simulink model "DA42HoloLensForwarder"  (R2021a)
settings: Solver=ode4  StartTime=0.0  StopTime=inf  FixedStep=0.001  RelTol=1e-3
undefined symbols (not defined in the file): Global_Sample_Time
libraries: simulink_extras x5, slrealtimeutilitieslib x2, dspnetwork x1
(part 1 of 5)
settings Model: EnablePacing=on  Creator=FCS Lab  LastModifiedBy=ga28nex
settings SolverCC: AlgebraicLoopSolver=TrustRegion
settings DebuggingCC: SFMachineParentedDataDiag=warning

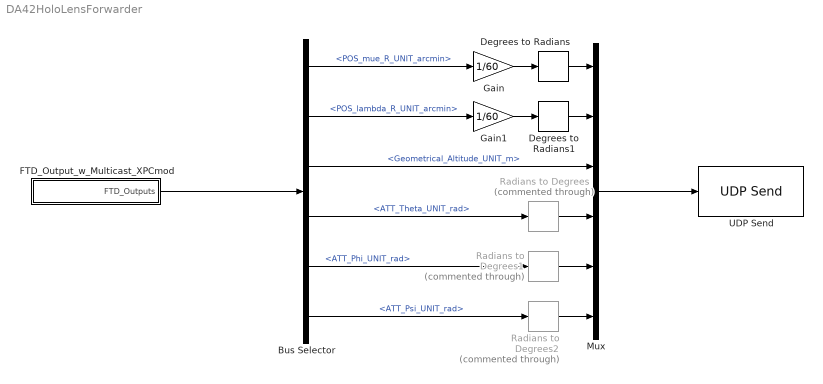
== system DA42HoloLensForwarder ==
  Bus Selector : BusSelector  OutputSignals=Host_Signals.POS_mue_R_UNIT_arcmin,Host_Signals.POS_lambda_R_UNIT_arcmin,Host_Signals.Geometrical_Altitude_UNIT_m,Host_Signals.ATT_Theta_UNIT_rad,Host_Signals.ATT_Phi_UNIT_rad,Host_Signals.ATT_Psi_UNIT_rad
  Degrees to Radians : simulink_extras/Transformations/Degrees to Radians
  Degrees to Radians1 : simulink_extras/Transformations/Degrees to Radians
  FTD_Output_w_Multicast_XPCmod : Subsystem
  Gain : Gain  Gain=1/60
  Gain1 : Gain  Gain=1/60
  Mux : Mux  Inputs=6
  Radians to Degrees : simulink_extras/Transformations/Radians to Degrees  Commented=through
  Radians to Degrees1 : simulink_extras/Transformations/Radians to Degrees  Commented=through
  Radians to Degrees2 : simulink_extras/Transformations/Radians to Degrees  Commented=through
  UDP Send : dspnetwork/UDP Send  remoteURL='127.0.0.1'  remotePort=53941  localURL='0.0.0.0'  localPortSource=Automatically determine  localPort=-1  sendBufferSize=8192  sampletime=-1  blockPlatform=[]  separateLengthPort=0
  wires:
  FTD_Output_w_Multicast_XPCmod/1(FTD_Outputs) -> Bus Selector/1
  Bus Selector/1 -> Gain/1  "<POS_mue_R_UNIT_arcmin>"
  Bus Selector/2 -> Gain1/1  "<POS_lambda_R_UNIT_arcmin>"
  Bus Selector/3 -> Mux/3  "<Geometrical_Altitude_UNIT_m>"
  Radians to Degrees/1 -> Mux/4
  Bus Selector/4 -> Radians to Degrees/1  "<ATT_Theta_UNIT_rad>"
  Radians to Degrees1/1 -> Mux/5
  Bus Selector/5 -> Radians to Degrees1/1  "<ATT_Phi_UNIT_rad>"
  Radians to Degrees2/1 -> Mux/6
  Bus Selector/6 -> Radians to Degrees2/1  "<ATT_Psi_UNIT_rad>"
  Mux/1 -> UDP Send/1
  Gain1/1 -> Degrees to Radians1/1
  Gain/1 -> Degrees to Radians/1
  Degrees to Radians/1 -> Mux/1
  Degrees to Radians1/1 -> Mux/2

== system DA42HoloLensForwarder/FTD_Output_w_Multicast_XPCmod ==
  Bus Creator : BusCreator  Inputs=3
  Hardware_Switches : Subsystem
  Host_Signals : Subsystem
  IO_Module_Pilot_Commands : Subsystem
  FTD_Outputs : Outport  BusOutputAsStruct=on
  wires:
  Bus Creator/1 -> FTD_Outputs/1  "FTD_Outputs"
  Host_Signals/1(Host_Signals) -> Bus Creator/1
  Hardware_Switches/1(Hardware_Switches) -> Bus Creator/3
  IO_Module_Pilot_Commands/1(Commands_Bus) -> Bus Creator/2
  IO_Module_Pilot_Commands/2(Switches) -> Hardware_Switches/1(Switches)

== system DA42HoloLensForwarder/FTD_Output_w_Multicast_XPCmod/Hardware_Switches ==
  note: CVCLVariable<double> MiscSwitches;
      | 	CVCLVariable<double> PanelAndLegroomSwitches;
      | 	CVCLVariable<double> SticksAndConsoleSwitches;
      | 	CVCLVariable<double> SticksDeviceConsoleSwitches;
  Switches : Inport
  Bus Creator2 : BusCreator  Inputs=3  NonVirtualBus=on
  Bus Selector : BusSelector  OutputSignals=MiscSwitches,PanelAndLegroomSwitches,SticksAndConsoleSwitches
  MiscSwitches : Subsystem
  PanelAndLegroomSwitches : Subsystem
  SticksAndConsoleSwitches : Subsystem
  Hardware_Switches : Outport
  wires:
  Bus Selector/2 -> PanelAndLegroomSwitches/1(PanelAndLegroomSwitches_MASK)  "<PanelAndLegroomSwitches>"
  Bus Selector/1 -> MiscSwitches/1(PanelAndLegroomSwitches_MASK)  "<MiscSwitches>"
  Bus Selector/3 -> SticksAndConsoleSwitches/1(PanelAndLegroomSwitches_MASK)  "<SticksAndConsoleSwitches>"
  PanelAndLegroomSwitches/1(PanelAndLegroomSwitches) -> Bus Creator2/2
  Bus Creator2/1 -> Hardware_Switches/1  "Hardware_Switches"
  MiscSwitches/1(MiscSwitches) -> Bus Creator2/1
  SticksAndConsoleSwitches/1(SticksAndConsoleSwitches) -> Bus Creator2/3
  Switches/1 -> Bus Selector/1

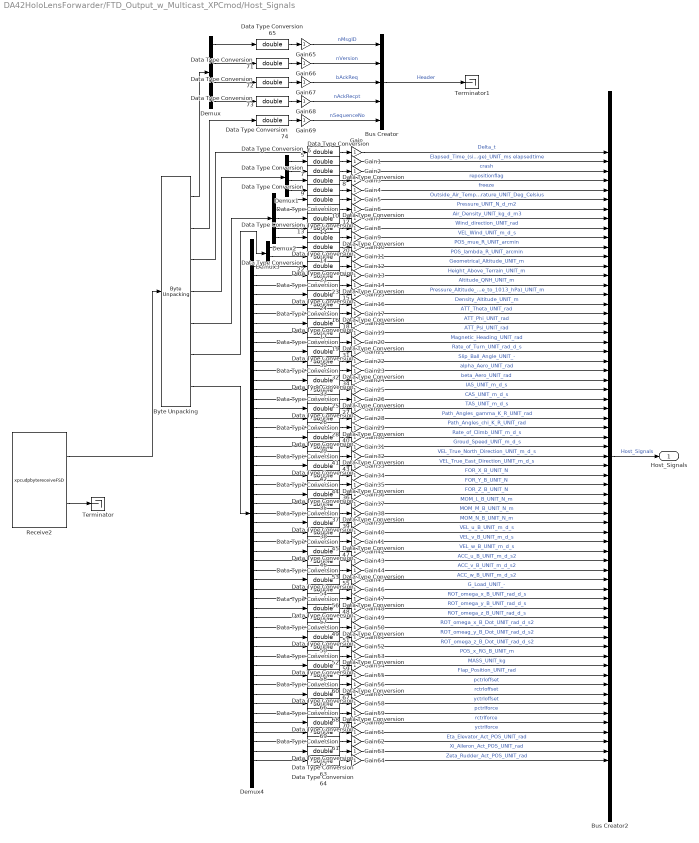
== system DA42HoloLensForwarder/FTD_Output_w_Multicast_XPCmod/Host_Signals ==
  Bus Creator : BusCreator  Inputs=5
  Bus Creator2 : BusCreator  Inputs=65  NonVirtualBus=on
  "Byte Unpacking " : slrealtimeutilitieslib/Byte Unpacking  MaskUnpackedDataTypes="{'uint8', 'uint32', 'single',  'uint32', 'single', 'double', 'single'}"  MaskUnpackedDataSizes={4, 1, 1, 4, 5, 2, 53}  MaskAlignment=1
      settings: SourceProductBaseCode=XP
  Data Type Conversion{5..74} (70 alike) : DataTypeConversion  OutDataTypeStr=double
  Demux : Demux
  Demux1 : Demux
  Demux2 : Demux  Outputs=5
  Demux3 : Demux  Outputs=2
  Demux4 : Demux  Outputs=53
  Gain{,1..69} (70 alike) : Gain
  Receive2 : S-Function  FunctionName=xpcudpbytereceiveFSD  Parameters=ipAdd, ipPort, width, sampletime, vblLen  SFunctionDeploymentMode=off  EnableBusSupport=off  mask(xpcudpbytereceive){ipAddress=234.1.1.2, ipPort=15150, width=276, vblLen=on, sampletime=Global_Sample_Time}
      mask prompts: ipAddress "IP address to receive from (0.0.0.0 for accepting all):"; ipPort "IP port to receive from:"; width "Output port width (number of bytes):"; vblLen "Allow variable length packets"; sampletime "Sample time:"
      mask init:
      | % mudp('ipPort', 'IP Port');
      | ipAdd = ipAddressFromString(ipAddress);
      mask Help: eval('xpcdoc(''UDP_Receive'')');
      mask Display: disp('FSD\nUDP-Receive\nBinary')
  Terminator : Terminator
  Terminator1 : Terminator
  Host_Signals : Outport
  wires:
  Receive2/2 -> Terminator/1
  Receive2/1 -> "Byte Unpacking "/1
  Gain64/1 -> Bus Creator2/65  "Zeta_Rudder_Act_POS_UNIT_rad"
  Gain63/1 -> Bus Creator2/64  "Xi_Aileron_Act_POS_UNIT_rad"
  Gain62/1 -> Bus Creator2/63  "Eta_Elevator_Act_POS_UNIT_rad"
  Gain61/1 -> Bus Creator2/62  "yctrlforce"
  Gain60/1 -> Bus Creator2/61  "rctrlforce"
  Gain59/1 -> Bus Creator2/60  "pctrlforce"
  Gain58/1 -> Bus Creator2/59  "yctrloffset"
  Gain57/1 -> Bus Creator2/58  "rctrloffset"
  Gain56/1 -> Bus Creator2/57  "pctrloffset"
  Gain55/1 -> Bus Creator2/56  "Flap_Position_UNIT_rad"
  Gain54/1 -> Bus Creator2/55  "MASS_UNIT_kg"
  Gain53/1 -> Bus Creator2/54  "POS_x_RG_B_UNIT_m"
  Gain52/1 -> Bus Creator2/53  "ROT_omega_z_B_Dot_UNIT_rad_d_s2"
  Gain51/1 -> Bus Creator2/52  "ROT_omeag_y_B_Dot_UNIT_rad_d_s2"
  Gain50/1 -> Bus Creator2/51  "ROT_omega_x_B_Dot_UNIT_rad_d_s2"
  Gain49/1 -> Bus Creator2/50  "ROT_omega_z_B_UNIT_rad_d_s"
  Gain48/1 -> Bus Creator2/49  "ROT_omega_y_B_UNIT_rad_d_s"
  Gain47/1 -> Bus Creator2/48  "ROT_omega_x_B_UNIT_rad_d_s"
  Gain46/1 -> Bus Creator2/47  "G_Load_UNIT_-"
  Gain45/1 -> Bus Creator2/46  "ACC_w_B_UNIT_m_d_s2"
  Gain44/1 -> Bus Creator2/45  "ACC_v_B_UNIT_m_d_s2"
  Gain43/1 -> Bus Creator2/44  "ACC_u_B_UNIT_m_d_s2"
  Gain42/1 -> Bus Creator2/43  "VEL_w_B_UNIT_m_d_s"
  Gain41/1 -> Bus Creator2/42  "VEL_v_B_UNIT_m_d_s"
  Gain40/1 -> Bus Creator2/41  "VEL_u_B_UNIT_m_d_s"
  Gain39/1 -> Bus Creator2/40  "MOM_N_B_UNIT_N_m"
  Gain38/1 -> Bus Creator2/39  "MOM_M_B_UNIT_N_m"
  Gain37/1 -> Bus Creator2/38  "MOM_L_B_UNIT_N_m"
  Gain36/1 -> Bus Creator2/37  "FOR_Z_B_UNIT_N"
  Gain35/1 -> Bus Creator2/36  "FOR_Y_B_UNIT_N"
  Gain34/1 -> Bus Creator2/35  "FOR_X_B_UNIT_N"
  Gain33/1 -> Bus Creator2/34  "VEL_True_East_Direction_UNIT_m_d_s"
  Gain32/1 -> Bus Creator2/33  "VEL_True_North_Direction_UNIT_m_d_s"
  Gain31/1 -> Bus Creator2/32  "Groud_Speed_UNIT_m_d_s"
  Gain30/1 -> Bus Creator2/31  "Rate_of_Climb_UNIT_m_d_s"
  Gain29/1 -> Bus Creator2/30  "Path_Angles_chi_K_R_UNIT_rad"
  Gain28/1 -> Bus Creator2/29  "Path_Angles_gamma_K_R_UNIT_rad"
  Gain27/1 -> Bus Creator2/28  "TAS_UNIT_m_d_s"
  Gain26/1 -> Bus Creator2/27  "CAS_UNIT_m_d_s"
  Gain25/1 -> Bus Creator2/26  "IAS_UNIT_m_d_s"
  Gain24/1 -> Bus Creator2/25  "beta_Aero_UNIT_rad"
  Bus Creator2/1 -> Host_Signals/1  "Host_Signals"
  Gain23/1 -> Bus Creator2/24  "alpha_Aero_UNIT_rad"
  Gain22/1 -> Bus Creator2/23  "Slip_Ball_Angle_UNIT_-"
  Gain21/1 -> Bus Creator2/22  "Rate_of_Turn_UNIT_rad_d_s"
  Gain20/1 -> Bus Creator2/21  "Magnetic_Heading_UNIT_rad"
  Gain19/1 -> Bus Creator2/20  "ATT_Psi_UNIT_rad"
  Gain18/1 -> Bus Creator2/19  "ATT_Phi_UNIT_rad"
  Gain17/1 -> Bus Creator2/18  "ATT_Theta_UNIT_rad"
  Gain16/1 -> Bus Creator2/17  "Density_Altitude_UNIT_m"
  Gain15/1 -> Bus Creator2/16  "Pressure_Altitude_(relative_to_1013_hPa)_UNIT_m"
  Gain14/1 -> Bus Creator2/15  "Altitude_QNH_UNIT_m"
  Gain13/1 -> Bus Creator2/14  "Height_Above_Terrain_UNIT_m"
  Gain12/1 -> Bus Creator2/13  "Geometrical_Altitude_UNIT_m"
  Gain11/1 -> Bus Creator2/12  "POS_lambda_R_UNIT_arcmin"
  Gain10/1 -> Bus Creator2/11  "POS_mue_R_UNIT_arcmin"
  Gain9/1 -> Bus Creator2/10  "VEL_Wind_UNIT_m_d_s"
  Gain8/1 -> Bus Creator2/9  "Wind_direction_UNIT_rad"
  Gain7/1 -> Bus Creator2/8  "Air_Density_UNIT_kg_d_m3"
  Gain6/1 -> Bus Creator2/7  "Pressure_UNIT_N_d_m2"
  Gain5/1 -> Bus Creator2/6  "Outside_Air_Temperature_UNIT_Deg_Celsius"
  Gain4/1 -> Bus Creator2/5  "freeze"
  Gain3/1 -> Bus Creator2/4  "repositionflag"
  Gain2/1 -> Bus Creator2/3  "crash"
  Gain1/1 -> Bus Creator2/2  "Elapsed_Time_(since_last_time_change)_UNIT_ms elapsedtime"
  Gain/1 -> Bus Creator2/1  "Delta_t"
  Data Type Conversion5/1 -> Gain/1
  Data Type Conversion6/1 -> Gain1/1
  Data Type Conversion7/1 -> Gain2/1
  Data Type Conversion8/1 -> Gain3/1
  Data Type Conversion9/1 -> Gain4/1
  Data Type Conversion10/1 -> Gain5/1
  Data Type Conversion11/1 -> Gain6/1
  Data Type Conversion12/1 -> Gain7/1
  Data Type Conversion13/1 -> Gain8/1
  Data Type Conversion14/1 -> Gain9/1
  Data Type Conversion20/1 -> Gain10/1
  Data Type Conversion21/1 -> Gain11/1
  Data Type Conversion22/1 -> Gain12/1
  Data Type Conversion23/1 -> Gain13/1
  Data Type Conversion24/1 -> Gain14/1
  Data Type Conversion15/1 -> Gain15/1
  Data Type Conversion16/1 -> Gain16/1
  Data Type Conversion17/1 -> Gain17/1
  Data Type Conversion18/1 -> Gain18/1
  Data Type Conversion19/1 -> Gain19/1
  Data Type Conversion30/1 -> Gain20/1
  Data Type Conversion31/1 -> Gain21/1
  Data Type Conversion32/1 -> Gain22/1
  Data Type Conversion33/1 -> Gain23/1
  Data Type Conversion34/1 -> Gain24/1
  Data Type Conversion25/1 -> Gain25/1
  Data Type Conversion26/1 -> Gain26/1
  Data Type Conversion27/1 -> Gain27/1
  Data Type Conversion28/1 -> Gain28/1
  Data Type Conversion29/1 -> Gain29/1
  Data Type Conversion40/1 -> Gain30/1
  Data Type Conversion41/1 -> Gain31/1
  Data Type Conversion42/1 -> Gain32/1
  Data Type Conversion43/1 -> Gain33/1
  Data Type Conversion44/1 -> Gain34/1
  Data Type Conversion35/1 -> Gain35/1
  Data Type Conversion36/1 -> Gain36/1
  Data Type Conversion37/1 -> Gain37/1
  Data Type Conversion38/1 -> Gain38/1
  Data Type Conversion39/1 -> Gain39/1
  Data Type Conversion45/1 -> Gain40/1
  Data Type Conversion46/1 -> Gain41/1
  Data Type Conversion47/1 -> Gain42/1
  Data Type Conversion53/1 -> Gain43/1
  Data Type Conversion54/1 -> Gain44/1
  Data Type Conversion55/1 -> Gain45/1
  Data Type Conversion56/1 -> Gain46/1
  Data Type Conversion57/1 -> Gain47/1
  Data Type Conversion48/1 -> Gain48/1
  Data Type Conversion49/1 -> Gain49/1
  Data Type Conversion50/1 -> Gain50/1
  Data Type Conversion51/1 -> Gain51/1
  Data Type Conversion52/1 -> Gain52/1
  Data Type Conversion58/1 -> Gain53/1
  Data Type Conversion59/1 -> Gain54/1
  Data Type Conversion60/1 -> Gain55/1
  Data Type Conversion66/1 -> Gain56/1
  Data Type Conversion67/1 -> Gain57/1
  Data Type Conversion68/1 -> Gain58/1
  Data Type Conversion69/1 -> Gain59/1
  Data Type Conversion70/1 -> Gain60/1
  Data Type Conversion61/1 -> Gain61/1
  Data Type Conversion62/1 -> Gain62/1
  Data Type Conversion63/1 -> Gain63/1
  Data Type Conversion64/1 -> Gain64/1
  "Byte Unpacking "/1 -> Demux/1
  "Byte Unpacking "/4 -> Demux1/1
  "Byte Unpacking "/5 -> Demux2/1
  "Byte Unpacking "/6 -> Demux3/1
  "Byte Unpacking "/7 -> Demux4/1
  Demux4/1 -> Data Type Conversion22/1
  Demux4/2 -> Data Type Conversion23/1
  Demux4/3 -> Data Type Conversion24/1
  Demux4/4 -> Data Type Conversion15/1
  Demux4/5 -> Data Type Conversion16/1
  Demux4/6 -> Data Type Conversion17/1
  Demux4/7 -> Data Type Conversion18/1
  Demux4/8 -> Data Type Conversion19/1
  Demux4/9 -> Data Type Conversion30/1
  Demux4/10 -> Data Type Conversion31/1
  Demux4/11 -> Data Type Conversion32/1
  Demux4/12 -> Data Type Conversion33/1
  Demux4/13 -> Data Type Conversion34/1
  Demux4/14 -> Data Type Conversion25/1
  Demux4/15 -> Data Type Conversion26/1
  Demux4/16 -> Data Type Conversion27/1
  Demux4/17 -> Data Type Conversion28/1
  Demux4/18 -> Data Type Conversion29/1
  Demux4/19 -> Data Type Conversion40/1
  Demux4/20 -> Data Type Conversion41/1
  Demux4/21 -> Data Type Conversion42/1
  Demux4/22 -> Data Type Conversion43/1
  Demux4/23 -> Data Type Conversion44/1
  Demux4/24 -> Data Type Conversion35/1
  Demux4/25 -> Data Type Conversion36/1
  Demux4/26 -> Data Type Conversion37/1
  Demux4/27 -> Data Type Conversion38/1
  Demux4/28 -> Data Type Conversion39/1
  Demux4/29 -> Data Type Conversion45/1
  Demux4/30 -> Data Type Conversion46/1
  Demux4/31 -> Data Type Conversion47/1
  Demux4/32 -> Data Type Conversion53/1
  Demux4/33 -> Data Type Conversion54/1
  Demux4/34 -> Data Type Conversion55/1
  Demux4/35 -> Data Type Conversion56/1
  Demux4/36 -> Data Type Conversion57/1
  Demux4/37 -> Data Type Conversion48/1
  Demux4/38 -> Data Type Conversion49/1
  Demux4/39 -> Data Type Conversion50/1
  Demux4/40 -> Data Type Conversion51/1
  Demux4/41 -> Data Type Conversion52/1
  Demux4/42 -> Data Type Conversion58/1
  Demux4/43 -> Data Type Conversion59/1
  Demux4/44 -> Data Type Conversion60/1
  Demux4/45 -> Data Type Conversion66/1
  Demux4/46 -> Data Type Conversion67/1
  Demux4/47 -> Data Type Conversion68/1
  Demux4/48 -> Data Type Conversion69/1
  Demux4/49 -> Data Type Conversion70/1
  Demux4/50 -> Data Type Conversion61/1
  Demux4/51 -> Data Type Conversion62/1
  Demux4/52 -> Data Type Conversion63/1
  Demux4/53 -> Data Type Conversion64/1
  Demux3/1 -> Data Type Conversion20/1
  Demux3/2 -> Data Type Conversion21/1
  Demux2/1 -> Data Type Conversion10/1
  Demux2/2 -> Data Type Conversion11/1
  Demux2/3 -> Data Type Conversion12/1
  Demux2/4 -> Data Type Conversion13/1
  Demux2/5 -> Data Type Conversion14/1
  Demux1/1 -> Data Type Conversion6/1
  Demux1/2 -> Data Type Conversion7/1
  Demux1/3 -> Data Type Conversion8/1
  Demux1/4 -> Data Type Conversion9/1
  "Byte Unpacking "/3 -> Data Type Conversion5/1
  Data Type Conversion65/1 -> Gain65/1
  Demux/1 -> Data Type Conversion65/1
  Data Type Conversion71/1 -> Gain66/1
  Demux/2 -> Data Type Conversion71/1
  Data Type Conversion73/1 -> Gain68/1
  Demux/3 -> Data Type Conversion72/1
  Demux/4 -> Data Type Conversion73/1
  "Byte Unpacking "/2 -> Data Type Conversion74/1
  Data Type Conversion74/1 -> Gain69/1
  Data Type Conversion72/1 -> Gain67/1
  Gain65/1 -> Bus Creator/1  "nMsgID"
  Gain66/1 -> Bus Creator/2  "nVersion"
  Gain67/1 -> Bus Creator/3  "bAckReq"
  Gain68/1 -> Bus Creator/4  "nAckRecpt"
  Gain69/1 -> Bus Creator/5  "nSequenceNo"
  Bus Creator/1 -> Terminator1/1  "Header"

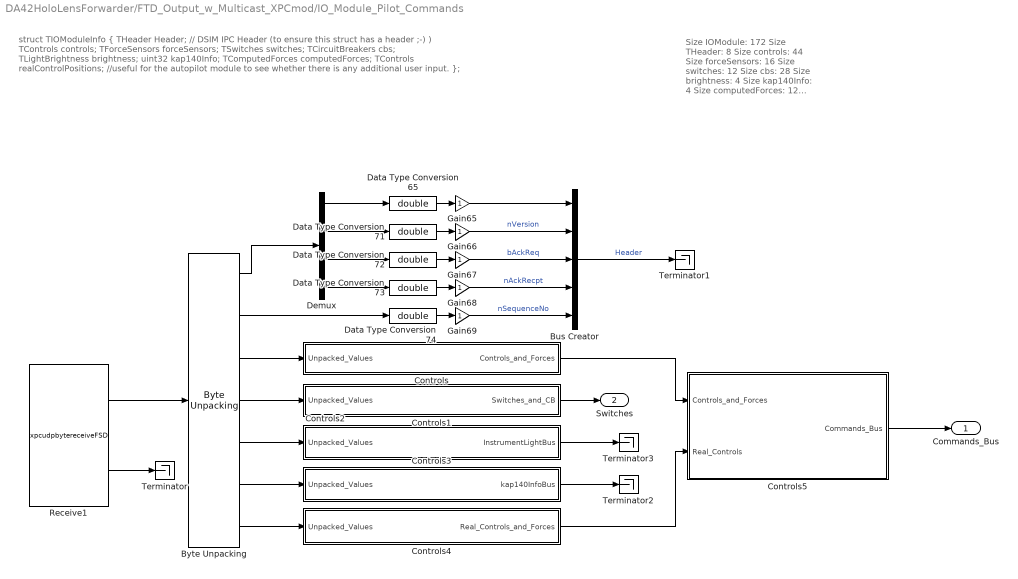
== system DA42HoloLensForwarder/FTD_Output_w_Multicast_XPCmod/IO_Module_Pilot_Commands ==
  note: Size IOModule: 172
      | Size THeader: 8
      | Size controls: 44
      | Size forceSensors: 16
      | Size switches: 12
      | Size cbs: 28
      | Size brightness: 4
      | Size kap140Info: 4
      | Size computedForces: 12
      | Size realControlPositions: 44
  note: struct TIOModuleInfo
      | {
      |     THeader             Header;     // DSIM IPC Header (to ensure this struct has a header ;-) )
      |     TControls           controls;
      |     TForceSensors       forceSensors;
      |     TSwitches           switches;
      |     TCircuitBreakers    cbs;
      |     TLightBrightness    brightness;
      |     uint32              kap140Info;
      |     TComputedForces     computedForces;
      |     TControls           realControlPositions; //useful for the autopilot module to see whether there is any additional user input.
      | };
  Bus Creator : BusCreator  Inputs=5
  "Byte Unpacking " : slrealtimeutilitieslib/Byte Unpacking  MaskUnpackedDataTypes="{'uint8', 'uint32', 'single',  'uint32', 'single', 'uint32', 'single'}"  MaskUnpackedDataSizes={4, 1, 15, 10, 1, 1, 14}  MaskAlignment=1
      settings: SourceProductBaseCode=XP
  Controls : Subsystem
  Controls1 : Subsystem
  Controls2 : Subsystem
  Controls3 : Subsystem
  Controls4 : Subsystem
  Controls5 : Subsystem
  Data Type Conversion{65,71..74} (5 alike) : DataTypeConversion  OutDataTypeStr=double
  Demux : Demux
  Gain{65..69} (5 alike) : Gain
  Receive1 : S-Function  FunctionName=xpcudpbytereceiveFSD  Parameters=ipAdd, ipPort, width, sampletime, vblLen  SFunctionDeploymentMode=off  EnableBusSupport=off  mask(xpcudpbytereceive){ipAddress=234.1.1.4, ipPort=15150, width=172, vblLen=on, sampletime=Global_Sample_Time}
      mask prompts: ipAddress "IP address to receive from (0.0.0.0 for accepting all):"; ipPort "IP port to receive from:"; width "Output port width (number of bytes):"; vblLen "Allow variable length packets"; sampletime "Sample time:"
      mask init:
      | % mudp('ipPort', 'IP Port');
      | ipAdd = ipAddressFromString(ipAddress);
      mask Help: eval('xpcdoc(''UDP_Receive'')');
      mask Display: disp('FSD\nUDP-Receive\nBinary')
  Terminator{,1..3} (4 alike) : Terminator
  Commands_Bus : Outport
  Switches : Outport  Port=2
  wires:
  Receive1/2 -> Terminator/1
  Receive1/1 -> "Byte Unpacking "/1
  Data Type Conversion71/1 -> Gain66/1
  Demux/2 -> Data Type Conversion71/1
  Data Type Conversion73/1 -> Gain68/1
  Demux/3 -> Data Type Conversion72/1
  Demux/4 -> Data Type Conversion73/1
  Data Type Conversion74/1 -> Gain69/1
  Data Type Conversion72/1 -> Gain67/1
  Gain66/1 -> Bus Creator/2  "nVersion"
  Gain67/1 -> Bus Creator/3  "bAckReq"
  Gain68/1 -> Bus Creator/4  "nAckRecpt"
  Gain69/1 -> Bus Creator/5  "nSequenceNo"
  Bus Creator/1 -> Terminator1/1  "Header"
  "Byte Unpacking "/1 -> Demux/1
  Demux/1 -> Data Type Conversion65/1
  Data Type Conversion65/1 -> Gain65/1
  Gain65/1 -> Bus Creator/1
  "Byte Unpacking "/2 -> Data Type Conversion74/1
  "Byte Unpacking "/3 -> Controls/1(Unpacked_Values)
  "Byte Unpacking "/4 -> Controls1/1(Unpacked_Values)
  "Byte Unpacking "/5 -> Controls2/1(Unpacked_Values)
  "Byte Unpacking "/6 -> Controls3/1(Unpacked_Values)
  "Byte Unpacking "/7 -> Controls4/1(Unpacked_Values)
  Controls/1(Controls_and_Forces) -> Controls5/1(Controls_and_Forces)
  Controls4/1(Real_Controls_and_Forces) -> Controls5/2(Real_Controls)
  Controls5/1(Commands_Bus) -> Commands_Bus/1
  Controls1/1(Switches_and_CB) -> Switches/1
  Controls3/1(kap140InfoBus) -> Terminator2/1
  Controls2/1(InstrumentLightBus) -> Terminator3/1

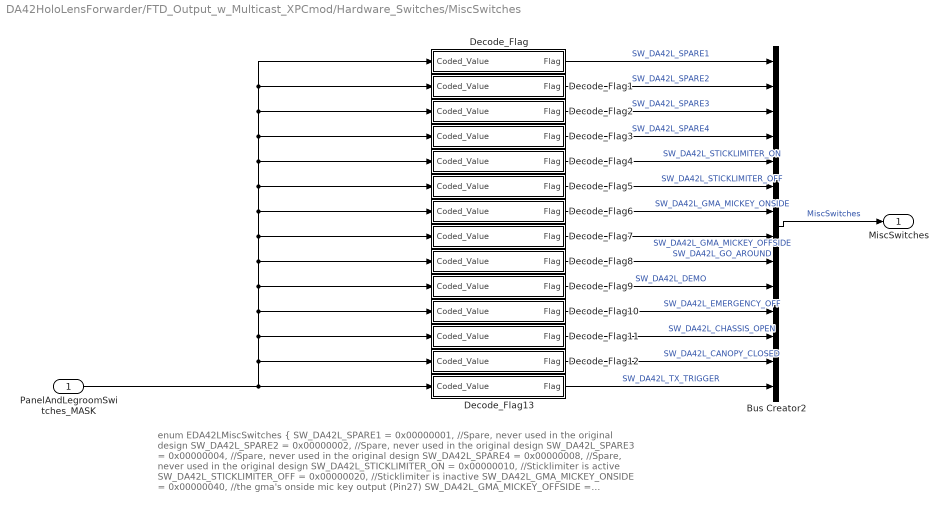
== system DA42HoloLensForwarder/FTD_Output_w_Multicast_XPCmod/Hardware_Switches/MiscSwitches ==
  note: enum EDA42LMiscSwitches
      | {
      |     SW_DA42L_SPARE1              = 0x00000001,    //Spare, never used in the original design
      |     SW_DA42L_SPARE2              = 0x00000002,    //Spare, never used in the original design
      |     SW_DA42L_SPARE3              = 0x00000004,    //Spare, never used in the original design
      |     SW_DA42L_SPARE4              = 0x00000008,    //Spare, never used in the original design
      |     SW_DA42L_STICKLIMITER_ON     = 0x00000010,    //Sticklimiter is active
      |     SW_DA42L_STICKLIMITER_OFF    = 0x00000020,    //Sticklimiter is inactive
      |     SW_DA42L_GMA_MICKEY_ONSIDE   = 0x00000040,    //the gma's onside mic key output (Pin27)
      |     SW_DA42L_GMA_MICKEY_OFFSIDE  = 0x00000080,    //the gma's offside mic key output (Pin33)
      |     SW_DA42L_GO_AROUND           = 0x00000100,    //Go Around for Autopilot
      |     SW_DA42L_DEMO                = 0x00000200,    //the demo-mode-switch (probably useless, but a nice, ready to be used and fully cabled spare ;-) )
      |     SW_DA42L_EMERGENCY_OFF       = 0x00000400,    //the big red emerg. off switch
      |     SW_DA42L_CHASSIS_OPEN        = 0x00000800,    //the chassis switch (proven to be useful as a spare... ;-) )
      |     SW_DA42L_CANOPY_CLOSED       = 0x00001000,    //canopy switch
      |     SW_DA42L_TX_TRIGGER          = 0x00002000     //external TX-trigger for the G1000
  PanelAndLegroomSwitches_MASK : Inport
  Bus Creator2 : BusCreator  Inputs=14  NonVirtualBus=on
  Decode_Flag : Subsystem  mask{Bitmask_Value='1'}
      mask prompts: Bitmask_Value "Bitmask (as an hex!!! value)"
  Decode_Flag1 : Subsystem  mask{Bitmask_Value='2'}
      mask prompts: Bitmask_Value "Bitmask (as an hex!!! value)"
  Decode_Flag10 : Subsystem  mask{Bitmask_Value='400'}
      mask prompts: Bitmask_Value "Bitmask (as an hex!!! value)"
  Decode_Flag11 : Subsystem  mask{Bitmask_Value='800'}
      mask prompts: Bitmask_Value "Bitmask (as an hex!!! value)"
  Decode_Flag12 : Subsystem  mask{Bitmask_Value='1000'}
      mask prompts: Bitmask_Value "Bitmask (as an hex!!! value)"
  Decode_Flag13 : Subsystem  mask{Bitmask_Value='2000'}
      mask prompts: Bitmask_Value "Bitmask (as an hex!!! value)"
  Decode_Flag2 : Subsystem  mask{Bitmask_Value='4'}
      mask prompts: Bitmask_Value "Bitmask (as an hex!!! value)"
  Decode_Flag3 : Subsystem  mask{Bitmask_Value='8'}
      mask prompts: Bitmask_Value "Bitmask (as an hex!!! value)"
  Decode_Flag4 : Subsystem  mask{Bitmask_Value='10'}
      mask prompts: Bitmask_Value "Bitmask (as an hex!!! value)"
  Decode_Flag5 : Subsystem  mask{Bitmask_Value='20'}
      mask prompts: Bitmask_Value "Bitmask (as an hex!!! value)"
  Decode_Flag6 : Subsystem  mask{Bitmask_Value='40'}
      mask prompts: Bitmask_Value "Bitmask (as an hex!!! value)"
  Decode_Flag7 : Subsystem  mask{Bitmask_Value='80'}
      mask prompts: Bitmask_Value "Bitmask (as an hex!!! value)"
  Decode_Flag8 : Subsystem  mask{Bitmask_Value='100'}
      mask prompts: Bitmask_Value "Bitmask (as an hex!!! value)"
  Decode_Flag9 : Subsystem  mask{Bitmask_Value='200'}
      mask prompts: Bitmask_Value "Bitmask (as an hex!!! value)"
  MiscSwitches : Outport
  wires:
  PanelAndLegroomSwitches_MASK/1 -> Decode_Flag13/1(Coded_Value), Decode_Flag12/1(Coded_Value), Decode_Flag11/1(Coded_Value), Decode_Flag10/1(Coded_Value), Decode_Flag9/1(Coded_Value), Decode_Flag8/1(Coded_Value), Decode_Flag7/1(Coded_Value), Decode_Flag6/1(Coded_Value), Decode_Flag5/1(Coded_Value), Decode_Flag4/1(Coded_Value), Decode_Flag3/1(Coded_Value), Decode_Flag2/1(Coded_Value), Decode_Flag1/1(Coded_Value), Decode_Flag/1(Coded_Value)
  Decode_Flag13/1(Flag) -> Bus Creator2/14  "SW_DA42L_TX_TRIGGER"
  Decode_Flag12/1(Flag) -> Bus Creator2/13  "SW_DA42L_CANOPY_CLOSED"
  Decode_Flag11/1(Flag) -> Bus Creator2/12  "SW_DA42L_CHASSIS_OPEN"
  Decode_Flag10/1(Flag) -> Bus Creator2/11  "SW_DA42L_EMERGENCY_OFF"
  Decode_Flag9/1(Flag) -> Bus Creator2/10  "SW_DA42L_DEMO"
  Decode_Flag8/1(Flag) -> Bus Creator2/9  "SW_DA42L_GO_AROUND"
  Decode_Flag7/1(Flag) -> Bus Creator2/8  "SW_DA42L_GMA_MICKEY_OFFSIDE"
  Decode_Flag6/1(Flag) -> Bus Creator2/7  "SW_DA42L_GMA_MICKEY_ONSIDE"
  Decode_Flag5/1(Flag) -> Bus Creator2/6  "SW_DA42L_STICKLIMITER_OFF"
  Decode_Flag4/1(Flag) -> Bus Creator2/5  "SW_DA42L_STICKLIMITER_ON"
  Decode_Flag3/1(Flag) -> Bus Creator2/4  "SW_DA42L_SPARE4"
  Decode_Flag2/1(Flag) -> Bus Creator2/3  "SW_DA42L_SPARE3"
  Decode_Flag1/1(Flag) -> Bus Creator2/2  "SW_DA42L_SPARE2"
  Decode_Flag/1(Flag) -> Bus Creator2/1  "SW_DA42L_SPARE1"
  Bus Creator2/1 -> MiscSwitches/1  "MiscSwitches"

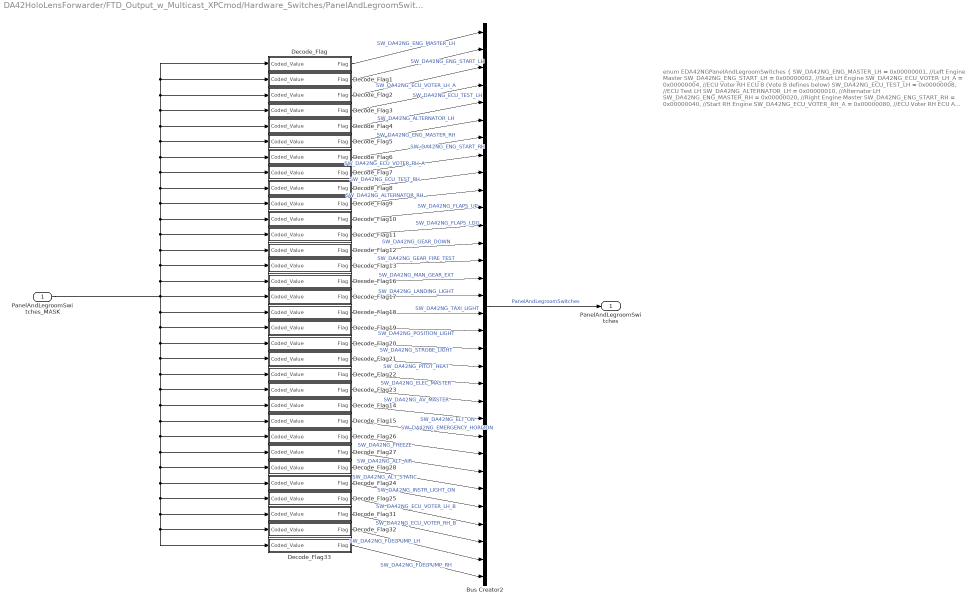
== system DA42HoloLensForwarder/FTD_Output_w_Multicast_XPCmod/Hardware_Switches/PanelAndLegroomSwitches ==
  note: enum EDA42NGPanelAndLegroomSwitches
      | {
      |     SW_DA42NG_ENG_MASTER_LH         =   0x00000001,     //Left Engine Master
      |     SW_DA42NG_ENG_START_LH          =   0x00000002,     //Start LH Engine
      |     SW_DA42NG_ECU_VOTER_LH_A        =   0x00000004,     //ECU Voter RH ECU B (Vote B defines below)
      |     SW_DA42NG_ECU_TEST_LH           =   0x00000008,     //ECU Test LH
      |     SW_DA42NG_ALTERNATOR_LH         =   0x00000010,     //Alternator LH
      |
      |     SW_DA42NG_ENG_MASTER_RH         =   0x00000020,     //Right Engine Master
      |     SW_DA42NG_ENG_START_RH          =   0x00000040,     //Start RH Engine
      |     SW_DA42NG_ECU_VOTER_RH_A        =   0x00000080,     //ECU Voter RH ECU A (Vote B defines below)
      |     SW_DA42NG_ECU_TEST_RH           =   0x00000100,     //ECU Test RH
      |     SW_DA42NG_ALTERNATOR_RH         =   0x00000200,     //Alternator RH
      |
      |     SW_DA42NG_FLAPS_UP              =   0x00000400,     //Flapswitch in position "Up"
      |     SW_DA42NG_FLAPS_LDG             =   0x00000800,     //Flapswitch in position "Ldg"
      |
      |     SW_DA42NG_GEAR_DOWN             =   0x00001000,     //gearlever in position "down"
      |     SW_DA42NG_GEAR_FIRE_TEST        =   0x00002000,     //Gear/Fire Test
      |     SW_DA42NG_MAN_GEAR_EXT          =   0x00004000,     //Manual Gear Ext.
      |
      |     SW_DA42NG_LANDING_LIGHT         =   0x00008000,     //landing light
      |     SW_DA42NG_TAXI_LIGHT            =   0x00010000,     //taxi light
      |     SW_DA42NG_POSITION_LIGHT        =   0x00020000,     //position light
      |     SW_DA42NG_STROBE_LIGHT          =   0x00040000,     //strobe light
      |
      |     SW_DA42NG_PITOT_HEAT            =   0x00080000,     //Pitot Heat
      |     SW_DA42NG_ELEC_MASTER           =   0x00100000,     //electrical master
      |     SW_DA42NG_AV_MASTER             =   0x00200000,     //avionic master
      |     SW_DA42NG_ELT_ON                =   0x00400000,     //ELT On
      |     SW_DA42NG_EMERGENCY_HORIZON     =   0x00800000,     //Emergency Horizon
      |     SW_DA42NG_FREEZE                =   0x01000000,     //the freeze switch (note: atm it's a push-button)
      |     SW_DA42NG_ALT_AIR               =   0x02000000,     //alt air
      |     SW_DA42NG_ALT_STATIC            =   0x04000000,     //Alt static
      |     SW_DA42NG_INSTR_LIGHT_ON        =   0x08000000,      //Instr. Light Dim Active
      |
      |     SW_DA42NG_ECU_VOTER_LH_B        =   0x10000000,    //ECU Voter LH ECU B
      |     SW_DA42NG_ECU_VOTER_RH_B        =   0x20000000,    //ECU Voter RH ECU B
      |     SW_DA42NG_FUELPUMP_LH           =   0x40000000,    //LH FuelPump
      |     SW_DA42NG_FUELPUMP_RH           =   0x80000000     //RH Fuelpump
  PanelAndLegroomSwitches_MASK : Inport
  Bus Creator2 : BusCreator  Inputs=32  NonVirtualBus=on
  Decode_Flag : Subsystem  mask{Bitmask_Value='1'}
      mask prompts: Bitmask_Value "Bitmask (as an hex!!! value)"
  Decode_Flag1 : Subsystem  mask{Bitmask_Value='2'}
      mask prompts: Bitmask_Value "Bitmask (as an hex!!! value)"
  Decode_Flag10 : Subsystem  mask{Bitmask_Value='400'}
      mask prompts: Bitmask_Value "Bitmask (as an hex!!! value)"
  Decode_Flag11 : Subsystem  mask{Bitmask_Value='800'}
      mask prompts: Bitmask_Value "Bitmask (as an hex!!! value)"
  Decode_Flag12 : Subsystem  mask{Bitmask_Value='1000'}
      mask prompts: Bitmask_Value "Bitmask (as an hex!!! value)"
  Decode_Flag13 : Subsystem  mask{Bitmask_Value='2000'}
      mask prompts: Bitmask_Value "Bitmask (as an hex!!! value)"
  Decode_Flag14 : Subsystem  mask{Bitmask_Value='400000'}
      mask prompts: Bitmask_Value "Bitmask (as an hex!!! value)"
  Decode_Flag15 : Subsystem  mask{Bitmask_Value='800000'}
      mask prompts: Bitmask_Value "Bitmask (as an hex!!! value)"
  Decode_Flag16 : Subsystem  mask{Bitmask_Value='4000'}
      mask prompts: Bitmask_Value "Bitmask (as an hex!!! value)"
  Decode_Flag17 : Subsystem  mask{Bitmask_Value='8000'}
      mask prompts: Bitmask_Value "Bitmask (as an hex!!! value)"
  Decode_Flag18 : Subsystem  mask{Bitmask_Value='10000'}
      mask prompts: Bitmask_Value "Bitmask (as an hex!!! value)"
  Decode_Flag19 : Subsystem  mask{Bitmask_Value='20000'}
      mask prompts: Bitmask_Value "Bitmask (as an hex!!! value)"
  Decode_Flag2 : Subsystem  mask{Bitmask_Value='4'}
      mask prompts: Bitmask_Value "Bitmask (as an hex!!! value)"
  Decode_Flag20 : Subsystem  mask{Bitmask_Value='40000'}
      mask prompts: Bitmask_Value "Bitmask (as an hex!!! value)"
  Decode_Flag21 : Subsystem  mask{Bitmask_Value='80000'}
      mask prompts: Bitmask_Value "Bitmask (as an hex!!! value)"
  Decode_Flag22 : Subsystem  mask{Bitmask_Value='100000'}
      mask prompts: Bitmask_Value "Bitmask (as an hex!!! value)"
  Decode_Flag23 : Subsystem  mask{Bitmask_Value='200000'}
      mask prompts: Bitmask_Value "Bitmask (as an hex!!! value)"
  Decode_Flag24 : Subsystem  mask{Bitmask_Value='800000'}
      mask prompts: Bitmask_Value "Bitmask (as an hex!!! value)"
  Decode_Flag25 : Subsystem  mask{Bitmask_Value='10000000'}
      mask prompts: Bitmask_Value "Bitmask (as an hex!!! value)"
  Decode_Flag26 : Subsystem  mask{Bitmask_Value='1000000'}
      mask prompts: Bitmask_Value "Bitmask (as an hex!!! value)"
  Decode_Flag27 : Subsystem  mask{Bitmask_Value='2000000'}
      mask prompts: Bitmask_Value "Bitmask (as an hex!!! value)"
  Decode_Flag28 : Subsystem  mask{Bitmask_Value='4000000'}
      mask prompts: Bitmask_Value "Bitmask (as an hex!!! value)"
  Decode_Flag3 : Subsystem  mask{Bitmask_Value='8'}
      mask prompts: Bitmask_Value "Bitmask (as an hex!!! value)"
  Decode_Flag31 : Subsystem  mask{Bitmask_Value='20000000'}
      mask prompts: Bitmask_Value "Bitmask (as an hex!!! value)"
  Decode_Flag32 : Subsystem  mask{Bitmask_Value='40000000'}
      mask prompts: Bitmask_Value "Bitmask (as an hex!!! value)"
  Decode_Flag33 : Subsystem  mask{Bitmask_Value='80000000'}
      mask prompts: Bitmask_Value "Bitmask (as an hex!!! value)"
  Decode_Flag4 : Subsystem  mask{Bitmask_Value='10'}
      mask prompts: Bitmask_Value "Bitmask (as an hex!!! value)"
  Decode_Flag5 : Subsystem  mask{Bitmask_Value='20'}
      mask prompts: Bitmask_Value "Bitmask (as an hex!!! value)"
  Decode_Flag6 : Subsystem  mask{Bitmask_Value='40'}
      mask prompts: Bitmask_Value "Bitmask (as an hex!!! value)"
  Decode_Flag7 : Subsystem  mask{Bitmask_Value='80'}
      mask prompts: Bitmask_Value "Bitmask (as an hex!!! value)"
  Decode_Flag8 : Subsystem  mask{Bitmask_Value='100'}
      mask prompts: Bitmask_Value "Bitmask (as an hex!!! value)"
  Decode_Flag9 : Subsystem  mask{Bitmask_Value='200'}
      mask prompts: Bitmask_Value "Bitmask (as an hex!!! value)"
  PanelAndLegroomSwitches : Outport
  wires:
  Bus Creator2/1 -> PanelAndLegroomSwitches/1  "PanelAndLegroomSwitches"
  Decode_Flag/1(Flag) -> Bus Creator2/1  "SW_DA42NG_ENG_MASTER_LH"
  Decode_Flag1/1(Flag) -> Bus Creator2/2  "SW_DA42NG_ENG_START_LH"
  Decode_Flag2/1(Flag) -> Bus Creator2/3  "SW_DA42NG_ECU_VOTER_LH_A"
  Decode_Flag3/1(Flag) -> Bus Creator2/4  "SW_DA42NG_ECU_TEST_LH"
  Decode_Flag4/1(Flag) -> Bus Creator2/5  "SW_DA42NG_ALTERNATOR_LH"
  Decode_Flag5/1(Flag) -> Bus Creator2/6  "SW_DA42NG_ENG_MASTER_RH"
  Decode_Flag6/1(Flag) -> Bus Creator2/7  "SW_DA42NG_ENG_START_RH"
  Decode_Flag7/1(Flag) -> Bus Creator2/8  "SW_DA42NG_ECU_VOTER_RH_A"
  Decode_Flag8/1(Flag) -> Bus Creator2/9  "SW_DA42NG_ECU_TEST_RH"
  Decode_Flag9/1(Flag) -> Bus Creator2/10  "SW_DA42NG_ALTERNATOR_RH"
  Decode_Flag10/1(Flag) -> Bus Creator2/11  "SW_DA42NG_FLAPS_UP"
  Decode_Flag11/1(Flag) -> Bus Creator2/12  "SW_DA42NG_FLAPS_LDG"
  Decode_Flag12/1(Flag) -> Bus Creator2/13  "SW_DA42NG_GEAR_DOWN"
  Decode_Flag13/1(Flag) -> Bus Creator2/14  "SW_DA42NG_GEAR_FIRE_TEST"
  Decode_Flag16/1(Flag) -> Bus Creator2/15  "SW_DA42NG_MAN_GEAR_EXT"
  Decode_Flag17/1(Flag) -> Bus Creator2/16  "SW_DA42NG_LANDING_LIGHT"
  Decode_Flag18/1(Flag) -> Bus Creator2/17  "SW_DA42NG_TAXI_LIGHT"
  Decode_Flag19/1(Flag) -> Bus Creator2/18  "SW_DA42NG_POSITION_LIGHT"
  Decode_Flag20/1(Flag) -> Bus Creator2/19  "SW_DA42NG_STROBE_LIGHT"
  Decode_Flag21/1(Flag) -> Bus Creator2/20  "SW_DA42NG_PITOT_HEAT"
  Decode_Flag22/1(Flag) -> Bus Creator2/21  "SW_DA42NG_ELEC_MASTER"
  Decode_Flag23/1(Flag) -> Bus Creator2/22  "SW_DA42NG_AV_MASTER"
  Decode_Flag14/1(Flag) -> Bus Creator2/23  "SW_DA42NG_ELT_ON"
  Decode_Flag15/1(Flag) -> Bus Creator2/24  "SW_DA42NG_EMERGENCY_HORIZON"
  Decode_Flag26/1(Flag) -> Bus Creator2/25  "SW_DA42NG_FREEZE"
  Decode_Flag27/1(Flag) -> Bus Creator2/26  "SW_DA42NG_ALT_AIR"
  Decode_Flag28/1(Flag) -> Bus Creator2/27  "SW_DA42NG_ALT_STATIC"
  Decode_Flag24/1(Flag) -> Bus Creator2/28  "SW_DA42NG_INSTR_LIGHT_ON"
  Decode_Flag25/1(Flag) -> Bus Creator2/29  "SW_DA42NG_ECU_VOTER_LH_B"
  Decode_Flag31/1(Flag) -> Bus Creator2/30  "SW_DA42NG_ECU_VOTER_RH_B"
  Decode_Flag32/1(Flag) -> Bus Creator2/31  "SW_DA42NG_FUELPUMP_LH"
  Decode_Flag33/1(Flag) -> Bus Creator2/32  "SW_DA42NG_FUELPUMP_RH"
  PanelAndLegroomSwitches_MASK/1 -> Decode_Flag17/1(Coded_Value), Decode_Flag/1(Coded_Value), Decode_Flag1/1(Coded_Value), Decode_Flag2/1(Coded_Value), Decode_Flag3/1(Coded_Value), Decode_Flag4/1(Coded_Value), Decode_Flag5/1(Coded_Value), Decode_Flag6/1(Coded_Value), Decode_Flag7/1(Coded_Value), Decode_Flag8/1(Coded_Value), Decode_Flag9/1(Coded_Value), Decode_Flag10/1(Coded_Value), Decode_Flag11/1(Coded_Value), Decode_Flag12/1(Coded_Value), Decode_Flag13/1(Coded_Value), Decode_Flag16/1(Coded_Value), Decode_Flag18/1(Coded_Value), Decode_Flag19/1(Coded_Value), Decode_Flag20/1(Coded_Value), Decode_Flag21/1(Coded_Value), Decode_Flag22/1(Coded_Value), Decode_Flag23/1(Coded_Value), Decode_Flag14/1(Coded_Value), Decode_Flag15/1(Coded_Value), Decode_Flag26/1(Coded_Value), Decode_Flag27/1(Coded_Value), Decode_Flag28/1(Coded_Value), Decode_Flag24/1(Coded_Value), Decode_Flag25/1(Coded_Value), Decode_Flag31/1(Coded_Value), Decode_Flag32/1(Coded_Value), Decode_Flag33/1(Coded_Value)

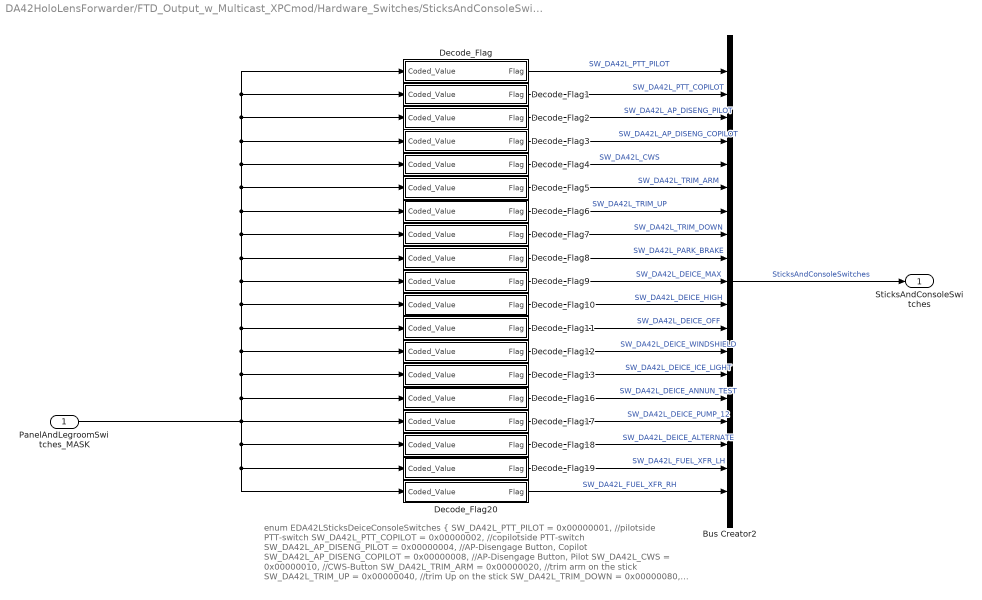
== system DA42HoloLensForwarder/FTD_Output_w_Multicast_XPCmod/Hardware_Switches/SticksAndConsoleSwitches ==
  note: enum EDA42LSticksDeiceConsoleSwitches
      | {
      |     SW_DA42L_PTT_PILOT          =   0x00000001,    //pilotside PTT-switch
      |     SW_DA42L_PTT_COPILOT        =   0x00000002,    //copilotside PTT-switch
      |     SW_DA42L_AP_DISENG_PILOT    =   0x00000004,    //AP-Disengage Button, Copilot
      |     SW_DA42L_AP_DISENG_COPILOT  =   0x00000008,    //AP-Disengage Button, Pilot
      |     SW_DA42L_CWS                =	0x00000010,    //CWS-Button
      |     SW_DA42L_TRIM_ARM           =   0x00000020,    //trim arm on the stick
      |     SW_DA42L_TRIM_UP            =   0x00000040,    //trim Up on the stick
      |     SW_DA42L_TRIM_DOWN          =   0x00000080,    //trim Down on the stick
      |     SW_DA42L_PARK_BRAKE         =	0x00000100,    //parking brake
      |     SW_DA42L_DEICE_MAX          =   0x00000200,    //MaxModeselect-pushbutton
      |     SW_DA42L_DEICE_HIGH         =   0x00000400,    //Modeselector switch
      |     SW_DA42L_DEICE_OFF          =   0x00000800,    //Modeselector switch
      |     SW_DA42L_DEICE_WINDSHIELD   =   0x00001000,    //Windshield-pushbutton
      |     SW_DA42L_DEICE_ICE_LIGHT    =   0x00002000,    //Icelight/off/Annuntest
      |     SW_DA42L_DEICE_ANNUN_TEST   =   0x00004000,    //Icelight/off/Annuntest
      |     SW_DA42L_DEICE_PUMP_12      =   0x00008000,    //0 selects pump1
      |     SW_DA42L_DEICE_ALTERNATE    =   0x00010000,     //Alternate Switch
      |     SW_DA42L_FUEL_XFR_LH        =   0x00020000,     //Fuel Transfer Switch for LH Aux Tank
      |     SW_DA42L_FUEL_XFR_RH        =   0x00040000      //Fuel Transfer Switch for RH Aux Tank
      |
      | };
  PanelAndLegroomSwitches_MASK : Inport
  Bus Creator2 : BusCreator  Inputs=19  NonVirtualBus=on
  Decode_Flag : Subsystem  mask{Bitmask_Value='1'}
      mask prompts: Bitmask_Value "Bitmask (as an hex!!! value)"
  Decode_Flag1 : Subsystem  mask{Bitmask_Value='2'}
      mask prompts: Bitmask_Value "Bitmask (as an hex!!! value)"
  Decode_Flag10 : Subsystem  mask{Bitmask_Value='400'}
      mask prompts: Bitmask_Value "Bitmask (as an hex!!! value)"
  Decode_Flag11 : Subsystem  mask{Bitmask_Value='800'}
      mask prompts: Bitmask_Value "Bitmask (as an hex!!! value)"
  Decode_Flag12 : Subsystem  mask{Bitmask_Value='1000'}
      mask prompts: Bitmask_Value "Bitmask (as an hex!!! value)"
  Decode_Flag13 : Subsystem  mask{Bitmask_Value='2000'}
      mask prompts: Bitmask_Value "Bitmask (as an hex!!! value)"
  Decode_Flag16 : Subsystem  mask{Bitmask_Value='4000'}
      mask prompts: Bitmask_Value "Bitmask (as an hex!!! value)"
  Decode_Flag17 : Subsystem  mask{Bitmask_Value='8000'}
      mask prompts: Bitmask_Value "Bitmask (as an hex!!! value)"
  Decode_Flag18 : Subsystem  mask{Bitmask_Value='10000'}
      mask prompts: Bitmask_Value "Bitmask (as an hex!!! value)"
  Decode_Flag19 : Subsystem  mask{Bitmask_Value='20000'}
      mask prompts: Bitmask_Value "Bitmask (as an hex!!! value)"
  Decode_Flag2 : Subsystem  mask{Bitmask_Value='4'}
      mask prompts: Bitmask_Value "Bitmask (as an hex!!! value)"
  Decode_Flag20 : Subsystem  mask{Bitmask_Value='40000'}
      mask prompts: Bitmask_Value "Bitmask (as an hex!!! value)"
  Decode_Flag3 : Subsystem  mask{Bitmask_Value='8'}
      mask prompts: Bitmask_Value "Bitmask (as an hex!!! value)"
  Decode_Flag4 : Subsystem  mask{Bitmask_Value='10'}
      mask prompts: Bitmask_Value "Bitmask (as an hex!!! value)"
  Decode_Flag5 : Subsystem  mask{Bitmask_Value='20'}
      mask prompts: Bitmask_Value "Bitmask (as an hex!!! value)"
  Decode_Flag6 : Subsystem  mask{Bitmask_Value='40'}
      mask prompts: Bitmask_Value "Bitmask (as an hex!!! value)"
  Decode_Flag7 : Subsystem  mask{Bitmask_Value='80'}
      mask prompts: Bitmask_Value "Bitmask (as an hex!!! value)"
  Decode_Flag8 : Subsystem  mask{Bitmask_Value='100'}
      mask prompts: Bitmask_Value "Bitmask (as an hex!!! value)"
  Decode_Flag9 : Subsystem  mask{Bitmask_Value='200'}
      mask prompts: Bitmask_Value "Bitmask (as an hex!!! value)"
  SticksAndConsoleSwitches : Outport
  wires:
  Bus Creator2/1 -> SticksAndConsoleSwitches/1  "SticksAndConsoleSwitches"
  Decode_Flag/1(Flag) -> Bus Creator2/1  "SW_DA42L_PTT_PILOT"
  Decode_Flag1/1(Flag) -> Bus Creator2/2  "SW_DA42L_PTT_COPILOT"
  Decode_Flag2/1(Flag) -> Bus Creator2/3  "SW_DA42L_AP_DISENG_PILOT"
  Decode_Flag3/1(Flag) -> Bus Creator2/4  "SW_DA42L_AP_DISENG_COPILOT"
  Decode_Flag4/1(Flag) -> Bus Creator2/5  "SW_DA42L_CWS"
  Decode_Flag5/1(Flag) -> Bus Creator2/6  "SW_DA42L_TRIM_ARM"
  Decode_Flag6/1(Flag) -> Bus Creator2/7  "SW_DA42L_TRIM_UP"
  Decode_Flag7/1(Flag) -> Bus Creator2/8  "SW_DA42L_TRIM_DOWN"
  Decode_Flag8/1(Flag) -> Bus Creator2/9  "SW_DA42L_PARK_BRAKE"
  Decode_Flag9/1(Flag) -> Bus Creator2/10  "SW_DA42L_DEICE_MAX"
  Decode_Flag10/1(Flag) -> Bus Creator2/11  "SW_DA42L_DEICE_HIGH"
  Decode_Flag11/1(Flag) -> Bus Creator2/12  "SW_DA42L_DEICE_OFF"
  Decode_Flag12/1(Flag) -> Bus Creator2/13  "SW_DA42L_DEICE_WINDSHIELD"
  Decode_Flag13/1(Flag) -> Bus Creator2/14  "SW_DA42L_DEICE_ICE_LIGHT"
  Decode_Flag16/1(Flag) -> Bus Creator2/15  "SW_DA42L_DEICE_ANNUN_TEST"
  Decode_Flag17/1(Flag) -> Bus Creator2/16  "SW_DA42L_DEICE_PUMP_12"
  Decode_Flag18/1(Flag) -> Bus Creator2/17  "SW_DA42L_DEICE_ALTERNATE"
  Decode_Flag19/1(Flag) -> Bus Creator2/18  "SW_DA42L_FUEL_XFR_LH"
  Decode_Flag20/1(Flag) -> Bus Creator2/19  "SW_DA42L_FUEL_XFR_RH"
  PanelAndLegroomSwitches_MASK/1 -> Decode_Flag17/1(Coded_Value), Decode_Flag/1(Coded_Value), Decode_Flag1/1(Coded_Value), Decode_Flag2/1(Coded_Value), Decode_Flag3/1(Coded_Value), Decode_Flag4/1(Coded_Value), Decode_Flag5/1(Coded_Value), Decode_Flag6/1(Coded_Value), Decode_Flag7/1(Coded_Value), Decode_Flag8/1(Coded_Value), Decode_Flag9/1(Coded_Value), Decode_Flag10/1(Coded_Value), Decode_Flag11/1(Coded_Value), Decode_Flag12/1(Coded_Value), Decode_Flag13/1(Coded_Value), Decode_Flag16/1(Coded_Value), Decode_Flag18/1(Coded_Value), Decode_Flag20/1(Coded_Value), Decode_Flag19/1(Coded_Value)

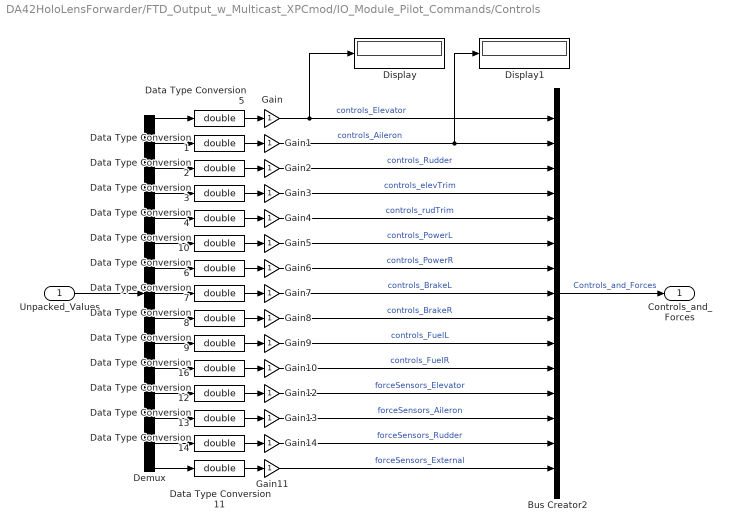
== system DA42HoloLensForwarder/FTD_Output_w_Multicast_XPCmod/IO_Module_Pilot_Commands/Controls ==
  Unpacked_Values : Inport
  Bus Creator2 : BusCreator  Inputs=15  NonVirtualBus=on
  Data Type Conversion{1..14,16} (15 alike) : DataTypeConversion  OutDataTypeStr=double
  Demux : Demux  Outputs=15
  Display : Display
  Display1 : Display
  Gain{,1..14} (15 alike) : Gain
  Controls_and_Forces : Outport
  wires:
  Gain10/1 -> Bus Creator2/11  "controls_FuelR"
  Gain9/1 -> Bus Creator2/10  "controls_FuelL"
  Gain8/1 -> Bus Creator2/9  "controls_BrakeR"
  Gain7/1 -> Bus Creator2/8  "controls_BrakeL"
  Gain6/1 -> Bus Creator2/7  "controls_PowerR"
  Gain5/1 -> Bus Creator2/6  "controls_PowerL"
  Gain4/1 -> Bus Creator2/5  "controls_rudTrim"
  Gain3/1 -> Bus Creator2/4  "controls_elevTrim"
  Gain2/1 -> Bus Creator2/3  "controls_Rudder"
  Gain1/1 -> Display1/1, Bus Creator2/2  "controls_Aileron"
  Gain/1 -> Display/1, Bus Creator2/1  "controls_Elevator"
  Data Type Conversion5/1 -> Gain/1
  Data Type Conversion1/1 -> Gain1/1
  Data Type Conversion2/1 -> Gain2/1
  Data Type Conversion3/1 -> Gain3/1
  Data Type Conversion4/1 -> Gain4/1
  Data Type Conversion6/1 -> Gain6/1
  Data Type Conversion7/1 -> Gain7/1
  Data Type Conversion8/1 -> Gain8/1
  Data Type Conversion9/1 -> Gain9/1
  Data Type Conversion10/1 -> Gain5/1
  Data Type Conversion16/1 -> Gain10/1
  Demux/1 -> Data Type Conversion5/1
  Demux/2 -> Data Type Conversion1/1
  Demux/3 -> Data Type Conversion2/1
  Demux/4 -> Data Type Conversion3/1
  Demux/5 -> Data Type Conversion4/1
  Demux/6 -> Data Type Conversion10/1
  Demux/7 -> Data Type Conversion6/1
  Demux/8 -> Data Type Conversion7/1
  Demux/9 -> Data Type Conversion8/1
  Demux/10 -> Data Type Conversion9/1
  Demux/11 -> Data Type Conversion16/1
  Data Type Conversion12/1 -> Gain12/1
  Data Type Conversion13/1 -> Gain13/1
  Data Type Conversion14/1 -> Gain14/1
  Data Type Conversion11/1 -> Gain11/1
  Gain12/1 -> Bus Creator2/12  "forceSensors_Elevator"
  Gain13/1 -> Bus Creator2/13  "forceSensors_Aileron"
  Gain14/1 -> Bus Creator2/14  "forceSensors_Rudder"
  Gain11/1 -> Bus Creator2/15  "forceSensors_External"
  Demux/12 -> Data Type Conversion12/1
  Demux/13 -> Data Type Conversion13/1
  Demux/14 -> Data Type Conversion14/1
  Demux/15 -> Data Type Conversion11/1
  Unpacked_Values/1 -> Demux/1
  Bus Creator2/1 -> Controls_and_Forces/1  "Controls_and_Forces"

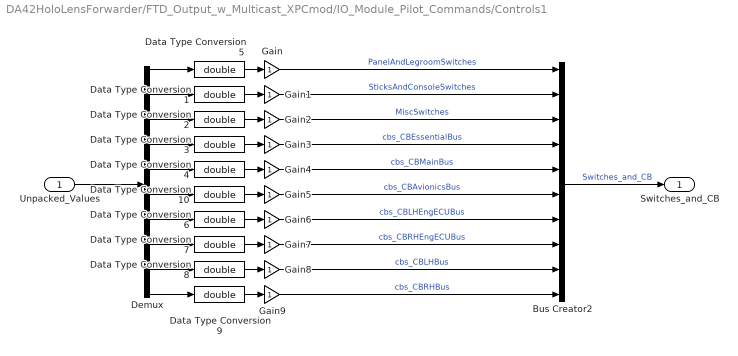
== system DA42HoloLensForwarder/FTD_Output_w_Multicast_XPCmod/IO_Module_Pilot_Commands/Controls1 ==
  Unpacked_Values : Inport
  Bus Creator2 : BusCreator  Inputs=10  NonVirtualBus=on
  Data Type Conversion{1..10} (10 alike) : DataTypeConversion  OutDataTypeStr=double
  Demux : Demux  Outputs=10
  Gain{,1..9} (10 alike) : Gain
  Switches_and_CB : Outport
  wires:
  Bus Creator2/1 -> Switches_and_CB/1  "Switches_and_CB"
  Unpacked_Values/1 -> Demux/1
  Demux/10 -> Data Type Conversion9/1
  Demux/9 -> Data Type Conversion8/1
  Demux/8 -> Data Type Conversion7/1
  Demux/7 -> Data Type Conversion6/1
  Demux/6 -> Data Type Conversion10/1
  Demux/5 -> Data Type Conversion4/1
  Demux/4 -> Data Type Conversion3/1
  Demux/3 -> Data Type Conversion2/1
  Demux/2 -> Data Type Conversion1/1
  Demux/1 -> Data Type Conversion5/1
  Data Type Conversion10/1 -> Gain5/1
  Data Type Conversion9/1 -> Gain9/1
  Data Type Conversion8/1 -> Gain8/1
  Data Type Conversion7/1 -> Gain7/1
  Data Type Conversion6/1 -> Gain6/1
  Data Type Conversion4/1 -> Gain4/1
  Data Type Conversion3/1 -> Gain3/1
  Data Type Conversion2/1 -> Gain2/1
  Data Type Conversion1/1 -> Gain1/1
  Data Type Conversion5/1 -> Gain/1
  Gain/1 -> Bus Creator2/1  "PanelAndLegroomSwitches"
  Gain1/1 -> Bus Creator2/2  "SticksAndConsoleSwitches"
  Gain2/1 -> Bus Creator2/3  "MiscSwitches"
  Gain3/1 -> Bus Creator2/4  "cbs_CBEssentialBus"
  Gain4/1 -> Bus Creator2/5  "cbs_CBMainBus"
  Gain5/1 -> Bus Creator2/6  "cbs_CBAvionicsBus"
  Gain6/1 -> Bus Creator2/7  "cbs_CBLHEngECUBus"
  Gain7/1 -> Bus Creator2/8  "cbs_CBRHEngECUBus"
  Gain8/1 -> Bus Creator2/9  "cbs_CBLHBus"
  Gain9/1 -> Bus Creator2/10  "cbs_CBRHBus"

== system DA42HoloLensForwarder/FTD_Output_w_Multicast_XPCmod/IO_Module_Pilot_Commands/Controls2 ==
  Unpacked_Values : Inport
  Bus Creator2 : BusCreator  Inputs=1  NonVirtualBus=on
  Data Type Conversion5 : DataTypeConversion  OutDataTypeStr=double
  Gain : Gain
  InstrumentLightBus : Outport
  wires:
  Gain/1 -> Bus Creator2/1  "InstrumentLight"
  Data Type Conversion5/1 -> Gain/1
  Unpacked_Values/1 -> Data Type Conversion5/1
  Bus Creator2/1 -> InstrumentLightBus/1  "InstrumentLightBus"

== system DA42HoloLensForwarder/FTD_Output_w_Multicast_XPCmod/IO_Module_Pilot_Commands/Controls3 ==
  Unpacked_Values : Inport
  Bus Creator2 : BusCreator  Inputs=1  NonVirtualBus=on
  Data Type Conversion5 : DataTypeConversion  OutDataTypeStr=double
  Gain : Gain
  kap140InfoBus : Outport
  wires:
  Bus Creator2/1 -> kap140InfoBus/1  "kap140InfoBus"
  Unpacked_Values/1 -> Data Type Conversion5/1
  Data Type Conversion5/1 -> Gain/1
  Gain/1 -> Bus Creator2/1  "kap140Info"

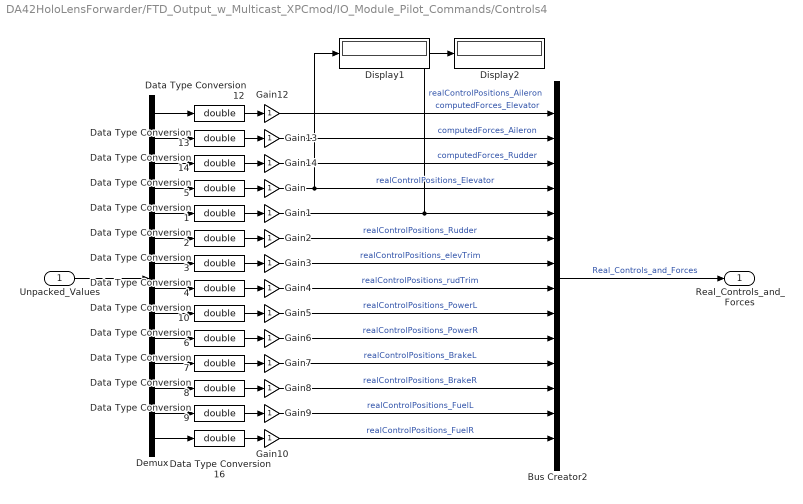
== system DA42HoloLensForwarder/FTD_Output_w_Multicast_XPCmod/IO_Module_Pilot_Commands/Controls4 ==
  Unpacked_Values : Inport
  Bus Creator2 : BusCreator  Inputs=14  NonVirtualBus=on
  Data Type Conversion{1..10,12..14,16} (14 alike) : DataTypeConversion  OutDataTypeStr=double
  Demux : Demux  Outputs=14
  Display1 : Display
  Display2 : Display
  Gain{,1..10,12..14} (14 alike) : Gain
  Real_Controls_and_Forces : Outport
  wires:
  Demux/14 -> Data Type Conversion16/1
  Demux/13 -> Data Type Conversion9/1
  Demux/12 -> Data Type Conversion8/1
  Demux/11 -> Data Type Conversion7/1
  Demux/10 -> Data Type Conversion6/1
  Demux/9 -> Data Type Conversion10/1
  Demux/8 -> Data Type Conversion4/1
  Demux/7 -> Data Type Conversion3/1
  Demux/6 -> Data Type Conversion2/1
  Demux/5 -> Data Type Conversion1/1
  Demux/4 -> Data Type Conversion5/1
  Demux/3 -> Data Type Conversion14/1
  Demux/2 -> Data Type Conversion13/1
  Demux/1 -> Data Type Conversion12/1
  Data Type Conversion12/1 -> Gain12/1
  Data Type Conversion13/1 -> Gain13/1
  Data Type Conversion14/1 -> Gain14/1
  Gain12/1 -> Bus Creator2/1  "computedForces_Elevator"
  Gain13/1 -> Bus Creator2/2  "computedForces_Aileron"
  Gain14/1 -> Bus Creator2/3  "computedForces_Rudder"
  Bus Creator2/1 -> Real_Controls_and_Forces/1  "Real_Controls_and_Forces"
  Unpacked_Values/1 -> Demux/1
  Data Type Conversion16/1 -> Gain10/1
  Data Type Conversion10/1 -> Gain5/1
  Data Type Conversion9/1 -> Gain9/1
  Data Type Conversion8/1 -> Gain8/1
  Data Type Conversion7/1 -> Gain7/1
  Data Type Conversion6/1 -> Gain6/1
  Data Type Conversion4/1 -> Gain4/1
  Data Type Conversion3/1 -> Gain3/1
  Data Type Conversion2/1 -> Gain2/1
  Data Type Conversion1/1 -> Gain1/1
  Data Type Conversion5/1 -> Gain/1
  Gain/1 -> Display1/1, Bus Creator2/4  "realControlPositions_Elevator"
  Gain1/1 -> Display2/1, Bus Creator2/5  "realControlPositions_Aileron"
  Gain2/1 -> Bus Creator2/6  "realControlPositions_Rudder"
  Gain3/1 -> Bus Creator2/7  "realControlPositions_elevTrim"
  Gain4/1 -> Bus Creator2/8  "realControlPositions_rudTrim"
  Gain5/1 -> Bus Creator2/9  "realControlPositions_PowerL"
  Gain6/1 -> Bus Creator2/10  "realControlPositions_PowerR"
  Gain7/1 -> Bus Creator2/11  "realControlPositions_BrakeL"
  Gain8/1 -> Bus Creator2/12  "realControlPositions_BrakeR"
  Gain9/1 -> Bus Creator2/13  "realControlPositions_FuelL"
  Gain10/1 -> Bus Creator2/14  "realControlPositions_FuelR"
